simulink model "SuperVoltageGenerator"  (R2024a)
settings: Solver=VariableStepAuto  StartTime=0.0  StopTime=5  RelTol=1e-3
libraries: spsSeriesRLCBranchLib x21, spsMosfetLib x15, spsVoltageMeasurementLib x8, simulink x6, spsDCVoltageSourceLib x3, spsDiodeLib x3, spsSawtoothGeneratorLib x3, spsGroundLib x1, spsLinearTransformerLib x1, sps_lib x1, dspstat3 x1
settings Model: Creator=Akbar  LastModifiedBy=Akbar

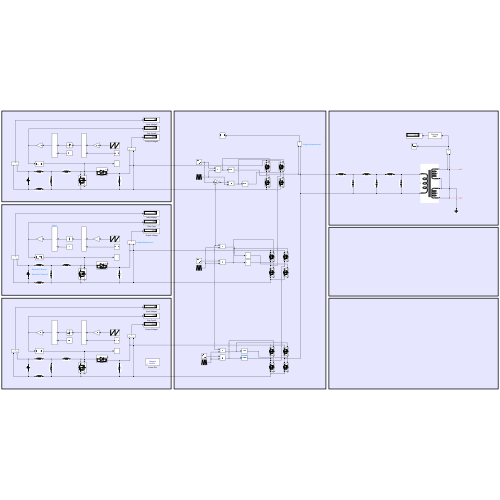
[thumbnail: Simulink's stored preview of the top-level diagram]
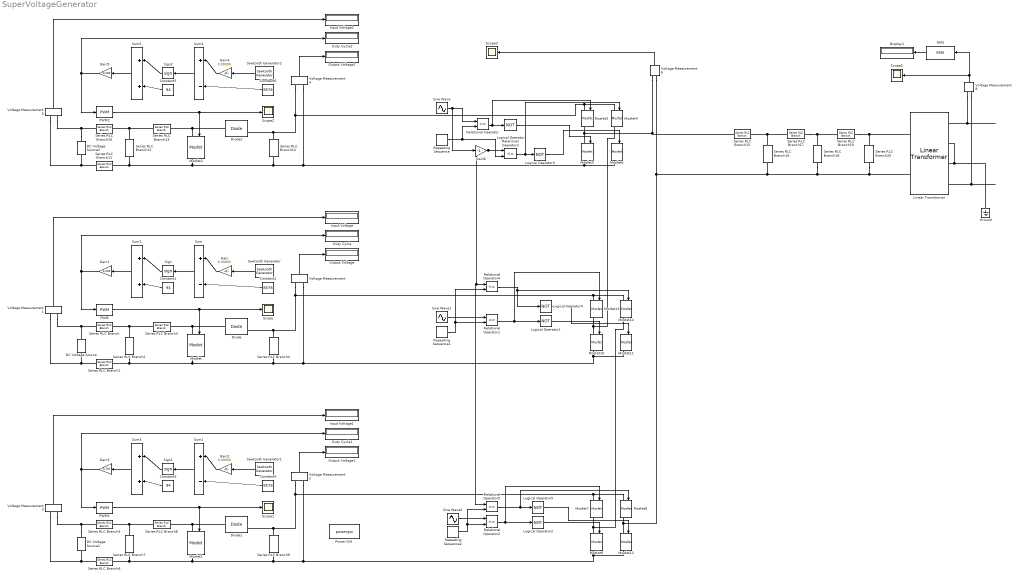
== system SuperVoltageGenerator ==
  Constant1 : Constant  Value=94
  Constant2 : Constant  Value=8576
  Constant3 : Constant  Value=94
  Constant4 : Constant  Value=8576
  Constant5 : Constant  Value=94
  Constant6 : Constant  Value=8576
  DC Voltage Source : spsDCVoltageSourceLib/DC Voltage Source  Amplitude=24  Measurements=None
  DC Voltage Source1 : spsDCVoltageSourceLib/DC Voltage Source  Amplitude=24  Measurements=None
  DC Voltage Source2 : spsDCVoltageSourceLib/DC Voltage Source  Amplitude=24  Measurements=None
  Diode : spsDiodeLib/Diode  Ron=0.001  Lon=0  Vf=0.8  IC=0  UseSnubber=0  Rs=500  Cs=250e-9  Measurements=on
  Diode1 : spsDiodeLib/Diode  Ron=0.001  Lon=0  Vf=0.8  IC=0  UseSnubber=0  Rs=500  Cs=250e-9  Measurements=on
  Diode2 : spsDiodeLib/Diode  Ron=0.001  Lon=0  Vf=0.8  IC=0  UseSnubber=0  Rs=500  Cs=250e-9  Measurements=on
  Display1 : Display
  Duty Cycle : Display
  Duty Cycle1 : Display
  Duty Cycle2 : Display
  Gain : Gain  Gain=0.00000
  Gain1 : Gain  Gain=1/100
  Gain2 : Gain  Gain=0.00000
  Gain3 : Gain  Gain=1/100
  Gain4 : Gain  Gain=0.00000
  Gain5 : Gain  Gain=1/100
  Gain6 : Gain  Gain=-1
  Ground : spsGroundLib/Ground  LConnTagsString=a
  Input Voltage : Display
  Input Voltage1 : Display
  Input Voltage2 : Display
  Linear Transformer : spsLinearTransformerLib/Linear Transformer  UNITS=pu  NominalPower=[ 250e6 60 ]  winding1=[7.35e+05 0.002 0.08]  winding2=[900.15e+05 0.002 0.08]  ThreeWindings=on  winding3=[900.15e+05 0.002 0.08]  RmLm=[499.98 500]  Measurements=None  DataType=off
  Logical Operator{,1..5} (6 alike) : Logic  Operator=NOT  AllPortsSameDT=off  OutDataTypeStr=boolean
  Mosfet{,1..14} (15 alike) : spsMosfetLib/Mosfet  Ron=0.1  Lon=0  Rd=0.01  Vfd=0  IC=0  Rs=1e5  Cs=inf  Measurements=on
  Output Voltage : Display
  Output Voltage1 : Display
  Output Voltage2 : Display
  PWM : simulink/Discontinuities/PWM  DisableCoverage=on  Period=1/100000  InitialDelay=0  DisallowZeroDutyCycle=off  RunAtFixedTimeIntervals=off  SampleTime=0.1
  PWM1 : simulink/Discontinuities/PWM  DisableCoverage=on  Period=1/100000  InitialDelay=0  DisallowZeroDutyCycle=off  RunAtFixedTimeIntervals=off  SampleTime=0.1
  PWM2 : simulink/Discontinuities/PWM  DisableCoverage=on  Period=1/100000  InitialDelay=0  DisallowZeroDutyCycle=off  RunAtFixedTimeIntervals=off  SampleTime=0.1
  Power GUI : sps_lib/powergui  Priority=1  SimulationMode=Discrete  SampleTime=50e-7  frequency=60  Iterations=50  frequencyindice=0  Pbase=100e6  ErrMax=1e-4  UnitsV=kV  UnitsW=MW  buscounter=0  FunctionMessages=off  echomessages=off  EnableUseOfTLC=off  CurrentSourceSwitches=off  DisableSnubberDevices=off  DisableRonSwitches=off  DisableVfSwitches=off  DisplayEquations=off  AutomaticDiscreteSolvers=off  SolverType=Tustin/Backward Euler (TBE)  Interpol=off  ExternalGateDelay=off  methode=off  Ts=100  x0status=blocks  SPID=on  SwTol=0  HookPort=off  NonlinearTolerance=1e-4  nMaxIteration=100  ContinueOnMaxIteration=off  RestoreLinks=warning  ResistiveCurrentMeasurement=off  Frange=[0:2:500]  Ylog=off  Xlog=on  ShowGrid=off  save=off  variable=ZData  structure=0  ZoomFFT=off  StartTime=0.0  cycles=1  DisplayStyle=1  fundamental=60  FreqAxis=off  MaxFrequency=1000  frequencyindicesteady=1  RmsSteady=1  display=off
  RMS : dspstat3/RMS  run=on  directionMode=Each column  dimension=1  InputProcessing=Columns as channels (frame based)  reset_popup=None
  Relational Operator{,1..5} (6 alike) : RelationalOperator  Operator=<=  OutDataTypeStr=boolean  RndMeth=Simplest  InputSameDT=off
  Repeating Sequence : simulink/Sources/Repeating Sequence  rep_seq_t=[0 0.5 1]/1000  rep_seq_y=[0 1 0]
  Repeating Sequence1 : simulink/Sources/Repeating Sequence  rep_seq_t=[0 0.5 1]/1000  rep_seq_y=[1 2 1]
  Repeating Sequence2 : simulink/Sources/Repeating Sequence  rep_seq_t=[0 0.5 1]/1000  rep_seq_y=[2 3 2]
  Sawtooth Generator : spsSawtoothGeneratorLib/Sawtooth Generator  Freq=25e3  Phase=0  Ts=0
  Sawtooth Generator1 : spsSawtoothGeneratorLib/Sawtooth Generator  Freq=25e3  Phase=0  Ts=0
  Sawtooth Generator2 : spsSawtoothGeneratorLib/Sawtooth Generator  Freq=25e3  Phase=0  Ts=0
  Scope{,1..3,5} (5 alike) : Scope
  Series RLC Branch{,1,5..6,10..11,15,17,19} (9 alike) : spsSeriesRLCBranchLib/Series RLC Branch  LConnTagsString=__new0  RConnTagsString=__new0  BranchType=L  Resistance=1  Inductance=1e-3  SetiL0=off  InitialCurrent=0  Capacitance=1e-6  Setx0=off  InitialVoltage=0  Measurements=None
  Series RLC Branch12 : spsSeriesRLCBranchLib/Series RLC Branch  LConnTagsString=__new0  RConnTagsString=__new0  BranchType=C  Resistance=1  Inductance=1e-3  SetiL0=off  InitialCurrent=0  Capacitance=1e-4  Setx0=off  InitialVoltage=0  Measurements=None
  Series RLC Branch13 : spsSeriesRLCBranchLib/Series RLC Branch  LConnTagsString=__new0  RConnTagsString=__new0  BranchType=L  Resistance=1  Inductance=75e-6  SetiL0=off  InitialCurrent=0  Capacitance=1e-6  Setx0=off  InitialVoltage=0  Measurements=None
  Series RLC Branch14 : spsSeriesRLCBranchLib/Series RLC Branch  LConnTagsString=__new0  RConnTagsString=__new0  BranchType=C  Resistance=1  Inductance=1e-3  SetiL0=off  InitialCurrent=0  Capacitance=1.2e-6  Setx0=off  InitialVoltage=0  Measurements=None
  Series RLC Branch16 : spsSeriesRLCBranchLib/Series RLC Branch  LConnTagsString=__new0  RConnTagsString=__new0  BranchType=C  Resistance=1  Inductance=1e-3  SetiL0=off  InitialCurrent=0  Capacitance=1e-2  Setx0=off  InitialVoltage=0  Measurements=None
  Series RLC Branch18 : spsSeriesRLCBranchLib/Series RLC Branch  LConnTagsString=__new0  RConnTagsString=__new0  BranchType=C  Resistance=1  Inductance=1e-3  SetiL0=off  InitialCurrent=0  Capacitance=1e-2  Setx0=off  InitialVoltage=0  Measurements=None
  Series RLC Branch2 : spsSeriesRLCBranchLib/Series RLC Branch  LConnTagsString=__new0  RConnTagsString=__new0  BranchType=C  Resistance=1  Inductance=1e-3  SetiL0=off  InitialCurrent=0  Capacitance=1e-4  Setx0=off  InitialVoltage=0  Measurements=None
  Series RLC Branch20 : spsSeriesRLCBranchLib/Series RLC Branch  LConnTagsString=__new0  RConnTagsString=__new0  BranchType=C  Resistance=1  Inductance=1e-3  SetiL0=off  InitialCurrent=0  Capacitance=1e-2  Setx0=off  InitialVoltage=0  Measurements=None
  Series RLC Branch3 : spsSeriesRLCBranchLib/Series RLC Branch  LConnTagsString=__new0  RConnTagsString=__new0  BranchType=L  Resistance=1  Inductance=75e-6  SetiL0=off  InitialCurrent=0  Capacitance=1e-6  Setx0=off  InitialVoltage=0  Measurements=None
  Series RLC Branch4 : spsSeriesRLCBranchLib/Series RLC Branch  LConnTagsString=__new0  RConnTagsString=__new0  BranchType=C  Resistance=1  Inductance=1e-3  SetiL0=off  InitialCurrent=0  Capacitance=1.2e-6  Setx0=off  InitialVoltage=0  Measurements=None
  Series RLC Branch7 : spsSeriesRLCBranchLib/Series RLC Branch  LConnTagsString=__new0  RConnTagsString=__new0  BranchType=C  Resistance=1  Inductance=1e-3  SetiL0=off  InitialCurrent=0  Capacitance=1e-4  Setx0=off  InitialVoltage=0  Measurements=None
  Series RLC Branch8 : spsSeriesRLCBranchLib/Series RLC Branch  LConnTagsString=__new0  RConnTagsString=__new0  BranchType=L  Resistance=1  Inductance=75e-6  SetiL0=off  InitialCurrent=0  Capacitance=1e-6  Setx0=off  InitialVoltage=0  Measurements=None
  Series RLC Branch9 : spsSeriesRLCBranchLib/Series RLC Branch  LConnTagsString=__new0  RConnTagsString=__new0  BranchType=C  Resistance=1  Inductance=1e-3  SetiL0=off  InitialCurrent=0  Capacitance=1.2e-6  Setx0=off  InitialVoltage=0  Measurements=None
  Sign : Signum
  Sign1 : Signum
  Sign2 : Signum
  Sine Wave : Sin  Amplitude=3  Frequency=314.15  SampleTime=0
  Sine Wave1 : Sin  Amplitude=3  Frequency=314.15  SampleTime=0
  Sine Wave2 : Sin  Amplitude=3  Frequency=314.15  SampleTime=0
  Sum : Sum  Inputs=|+-
  Sum1 : Sum  Inputs=|++
  Sum2 : Sum  Inputs=|+-
  Sum3 : Sum  Inputs=|++
  Sum4 : Sum  Inputs=|+-
  Sum5 : Sum  Inputs=|++
  Voltage Measurement{,1..6,8} (8 alike) : spsVoltageMeasurementLib/Voltage Measurement  PhasorSimulation=off  OutputType=Complex  PSBequivalent=0
  wires:
  Constant1/1 -> Sum1/2
  Sawtooth Generator/1 -> Gain/1
  Sum/1 -> Sign/1
  Constant2/1 -> Sum/2
  Sign/1 -> Sum1/1
  Gain/1 -> Sum/1
  PWM/1 -> Mosfet/1, Scope/1
  Sum1/1 -> Gain1/1
  Gain1/1 -> PWM/1, Duty Cycle/1
  Voltage Measurement/1 -> Output Voltage/1
  Voltage Measurement1/1 -> Input Voltage/1
  Gain3/1 -> PWM1/1, Duty Cycle1/1
  Sum3/1 -> Gain3/1
  Constant4/1 -> Sum2/2
  PWM1/1 -> Mosfet1/1, Scope1/1
  Voltage Measurement2/1 -> Output Voltage1/1
  Sign1/1 -> Sum3/1
  Gain2/1 -> Sum2/1
  Constant3/1 -> Sum3/2
  Sawtooth Generator1/1 -> Gain2/1
  Sum2/1 -> Sign1/1
  Voltage Measurement3/1 -> Input Voltage1/1
  Gain5/1 -> PWM2/1, Duty Cycle2/1
  Sum5/1 -> Gain5/1
  Constant6/1 -> Sum4/2
  PWM2/1 -> Mosfet2/1, Scope2/1
  Voltage Measurement4/1 -> Output Voltage2/1
  Sign2/1 -> Sum5/1
  Gain4/1 -> Sum4/1
  Constant5/1 -> Sum5/2
  Sawtooth Generator2/1 -> Gain4/1
  Sum4/1 -> Sign2/1
  Voltage Measurement5/1 -> Input Voltage2/1
  Relational Operator4/1 -> Mosfet14/1, Logical Operator4/1
  Repeating Sequence2/1 -> Relational Operator5/2, Relational Operator2/2
  Logical Operator4/1 -> Mosfet11/1
  Logical Operator2/1 -> Mosfet9/1
  Relational Operator5/1 -> Mosfet8/1, Logical Operator5/1
  Logical Operator3/1 -> Mosfet6/1
  Relational Operator3/1 -> Mosfet4/1, Logical Operator3/1
  Gain6/1 -> Relational Operator3/1, Relational Operator5/1, Relational Operator4/1
  Logical Operator5/1 -> Mosfet12/1
  Logical Operator1/1 -> Mosfet10/1
  Repeating Sequence1/1 -> Relational Operator4/2, Relational Operator1/2
  Voltage Measurement6/1 -> Scope3/1
  Relational Operator2/1 -> Mosfet7/1, Logical Operator2/1
  Sine Wave1/1 -> Relational Operator1/1
  Relational Operator1/1 -> Mosfet13/1, Logical Operator1/1
  Repeating Sequence/1 -> Relational Operator3/2, Relational Operator/2
  Logical Operator/1 -> Mosfet5/1
  Sine Wave2/1 -> Relational Operator2/1
  Relational Operator/1 -> Mosfet3/1, Logical Operator/1
  Sine Wave/1 -> Gain6/1, Relational Operator/1
  Voltage Measurement8/1 -> RMS/1, Scope5/1
  RMS/1 -> Display1/1
  connections:
  Series RLC Branch/LConn1 -- Voltage Measurement1/LConn1 -- DC Voltage Source/RConn1
  Series RLC Branch1/RConn1 -- Voltage Measurement1/LConn2 -- DC Voltage Source/LConn1
  Series RLC Branch2/LConn1 -- Series RLC Branch3/LConn1 -- Series RLC Branch/RConn1
  Mosfet10/RConn1 -- Mosfet/RConn1 -- Series RLC Branch2/RConn1 -- Series RLC Branch1/LConn1 -- Series RLC Branch4/RConn1 -- Voltage Measurement/LConn2 -- Mosfet11/RConn1
  Mosfet/LConn1 -- Diode/LConn1 -- Series RLC Branch3/RConn1
  Mosfet13/LConn1 -- Diode/RConn1 -- Series RLC Branch4/LConn1 -- Voltage Measurement/LConn1 -- Mosfet14/LConn1
  Series RLC Branch6/RConn1 -- Voltage Measurement3/LConn2 -- DC Voltage Source1/LConn1
  DC Voltage Source1/RConn1 -- Series RLC Branch5/LConn1 -- Voltage Measurement3/LConn1
  Mosfet12/RConn1 -- Voltage Measurement2/LConn2 -- Mosfet1/RConn1 -- Series RLC Branch7/RConn1 -- Series RLC Branch6/LConn1 -- Series RLC Branch9/RConn1 -- Mosfet9/RConn1
  Mosfet8/LConn1 -- Diode1/RConn1 -- Series RLC Branch9/LConn1 -- Voltage Measurement2/LConn1 -- Mosfet7/LConn1
  Series RLC Branch5/RConn1 -- Series RLC Branch8/LConn1 -- Series RLC Branch7/LConn1
  Series RLC Branch8/RConn1 -- Mosfet1/LConn1 -- Diode1/LConn1
  Series RLC Branch11/RConn1 -- Voltage Measurement5/LConn2 -- DC Voltage Source2/LConn1
  DC Voltage Source2/RConn1 -- Series RLC Branch10/LConn1 -- Voltage Measurement5/LConn1
  Mosfet6/RConn1 -- Voltage Measurement4/LConn2 -- Mosfet2/RConn1 -- Series RLC Branch12/RConn1 -- Series RLC Branch11/LConn1 -- Series RLC Branch14/RConn1 -- Mosfet5/RConn1
  Mosfet4/LConn1 -- Voltage Measurement4/LConn1 -- Diode2/RConn1 -- Series RLC Branch14/LConn1 -- Mosfet3/LConn1
  Series RLC Branch10/RConn1 -- Series RLC Branch13/LConn1 -- Series RLC Branch12/LConn1
  Series RLC Branch13/RConn1 -- Mosfet2/LConn1 -- Diode2/LConn1
  Voltage Measurement6/LConn2 -- Linear Transformer/LConn2 -- Series RLC Branch20/RConn1 -- Series RLC Branch18/RConn1 -- Series RLC Branch16/RConn1 -- Mosfet12/LConn1 -- Mosfet8/RConn1
  Mosfet10/LConn1 -- Mosfet13/RConn1 -- Mosfet4/RConn1
  Mosfet9/LConn1 -- Mosfet7/RConn1 -- Mosfet14/RConn1
  Series RLC Branch15/LConn1 -- Mosfet3/RConn1 -- Mosfet5/LConn1 -- Voltage Measurement6/LConn1
  Series RLC Branch15/RConn1 -- Series RLC Branch17/LConn1 -- Series RLC Branch16/LConn1
  Series RLC Branch18/LConn1 -- Series RLC Branch17/RConn1 -- Series RLC Branch19/LConn1
  Series RLC Branch20/LConn1 -- Linear Transformer/LConn1 -- Series RLC Branch19/RConn1
  Linear Transformer/RConn3 -- Ground/LConn1 -- Linear Transformer/RConn2
  Voltage Measurement8/LConn1 -- Linear Transformer/RConn1
  Voltage Measurement8/LConn2 -- Linear Transformer/RConn4
